simulink model "EV_basic_8_1"  (R2018b)
settings: Solver=VariableStepAuto  StartTime=0.0  StopTime=950  MaxStep=1e-2  MinStep=1e-4  RelTol=1e-2
values from neighbouring files (symbols this model uses):
  Av = 2.75    [InitiateModel.m]    (also in InitiateModel_layouts.m; nurburg_lap.mat)
  batt_max_v = cell_series*cell_max_v    [InitiateModel.m]    (also in nurburg_lap.mat = 613.2)
  Capacity = batt_cap*1e3*3600    (= 252000000)    [InitiateModel.m]    (also in InitiateModel_layouts.m = 252000; nurburg_lap.mat = 180000000)
  Cd = 0.26    [InitiateModel.m]    (also in InitiateModel_layouts.m; nurburg_lap.mat)
  Cr = 0.01    [InitiateModel.m]    (also in InitiateModel_layouts.m; nurburg_lap.mat)
  eta_DC = .985    (= 0.985)    [InitiateModel.m]    (also in InitiateModel_layouts.m; nurburg_lap.mat)
  eta_inv = .965    (= 0.965)    [InitiateModel.m]    (also in InitiateModel_layouts.m; nurburg_lap.mat)
  front_motor = 2    [InitiateModel.m]    (also in nurburg_lap.mat = 0)
  Fv_max = 2*Fv_max_electric    (= 22377.6223776)    [InitiateModel.m]    (also in InitiateModel_layouts.m = 16783.2167832; nurburg_lap.mat)
  Fz_tire = (Mv * weight_dist * 0.5)*9.81    [InitiateModel.m]    (also in nurburg_lap.mat = 5290.7414625)
  gratio = 7    [InitiateModel.m]    (also in InitiateModel_layouts.m = 5.3; nurburg_lap.mat = 5.5)
  grav = 9.81    [InitiateModel.m]    (also in InitiateModel_layouts.m; nurburg_lap.mat)
  inv_eff = 0.98    [InitiateModel.m]    (also in nurburg_lap.mat)
  Ke = 0.607    [InitiateModel.m]    (also in InitiateModel_layouts.m; nurburg_lap.mat)
  max_curr = cell_max_curr*cells_parallel    [InitiateModel.m]    (also in InitiateModel_layouts.m = 270; nurburg_lap.mat = 400)
  motoreff_T = linspace(0,300,101)    [InitiateModel.m]    (also in motoreff_w.mat = [0 4 8 12 16 20 24 28 32 36 40 44 ... (101 elements, 1x101)]; nurburg_lap.mat = [0 3 6 9 12 15 18 21 24 27 30 33 ... (101 elements, 1x101)])
  motoreff_w = [0 18 36 54 72 90 108 126 144 162 180 198 ... (101 elements, 1x101)]    [motoreff_w.mat]    (also in nurburg_lap.mat = [0 12 24 36 48 60 72 84 96 108 120 132 ... (101 elements, 1x)
  Mv = 1420    [InitiateModel.m]    (also in InitiateModel_layouts.m; nurburg_lap.mat)
  opt_slip = 0.18    [InitiateModel.m]    (also in nurburg_lap.mat)
  Pe_max = 160e3    (= 160000)    [InitiateModel.m]    (also in InitiateModel_layouts.m = 120000; nurburg_lap.mat)
  rear_motor = 2    [InitiateModel.m]    (also in nurburg_lap.mat)
  regen_eff = 0.8    [InitiateModel.m]    (also in nurburg_lap.mat)
  rho_air = 1.204    [InitiateModel.m]    (also in InitiateModel_layouts.m; nurburg_lap.mat)
  rw = 0.668/2    (= 0.334)    [InitiateModel.m]    (also in InitiateModel_layouts.m; nurburg_lap.mat)
  s_time = 0.01    [InitiateModel.m]    (also in InitiateModel_layouts.m; nurburg_lap.mat)
  SOC_0 = 80    [InitiateModel.m]    (also in InitiateModel_layouts.m; nurburg_lap.mat)
  Te_max = 2*Te_max_electric    (= 2442.52479547)    [InitiateModel.m]    (also in InitiateModel_layouts.m = 1831.8935966; nurburg_lap.mat)
  tstep = .01    (= 0.01)    [InitiateModel.m]    (also in InitiateModel_layouts.m; nurburg_lap.mat)
  Vbase = 14.30    (= 14.3)    [InitiateModel.m]    (also in InitiateModel_layouts.m; nurburg_lap.mat)
  Vbus_ref = 600    [InitiateModel.m]    (also in InitiateModel_layouts.m = 530; nurburg_lap.mat)
  W_d = 0.5    [InitiateModel.m]    (also in InitiateModel_layouts.m; nurburg_lap.mat)
undefined symbols (not defined in the file or in its folder): MException, throw
libraries: simulink x6, autolibshared x3, peGeneralControl x1, autolibdcdc x1
(part 1 of 4)
settings Model: PacingRate=112  Creator=ignaciovicente  LastModifiedBy=htpc
settings SolverCC: ZeroCrossAlgorithm=Adaptive
settings OptimizationCC: EfficientMapNaN2IntZero=off
settings DebuggingCC: MaskedZcDiagnostic=none  IgnoredZcDiagnostic=none  LibraryContextMissingDiagnostic=none
settings HardwareCC: ProdBitPerLong=64  ProdHWDeviceType=Intel->x86-64 (Mac OS X)  TargetBitPerPointer=64  TargetBitPerSizeT=64  TargetBitPerPtrDiffT=64  TargetLongLongMode=on  TargetIntDivRoundTo=Zero  TargetEndianess=LittleEndian  TargetWordSize=64  TargetHWDeviceType=MATLAB Host  ProdEqTarget=off
settings SFSimCC: SimUseLocalCustomCode=off
settings CodeAppCC: MaxIdLength=128
settings GRTTargetCC: TargetLangStandard=C89/C90 (ANSI)  CombineOutputUpdateFcns=off  GRTInterface=on

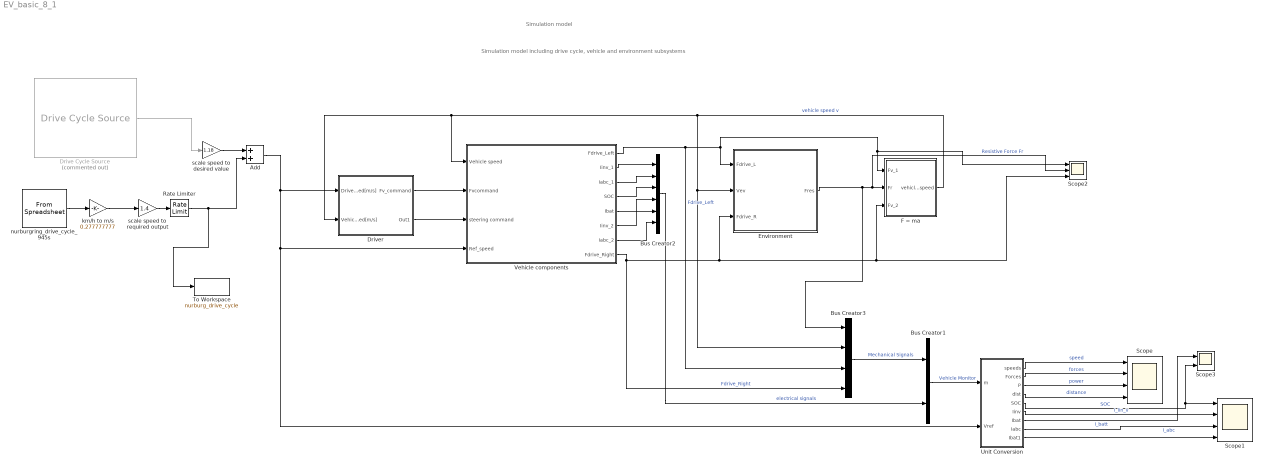
== system EV_basic_8_1 ==
  note: Simulation model including drive cycle, vehicle and environment subsystems
  note: Simulation model
  Add : Sum
  Bus Creator1 : BusCreator  Inputs=2
  Bus Creator2 : BusCreator  Inputs=6
  Bus Creator3 : BusCreator  Inputs=4
  Drive Cycle Source : autolibshared/Drive Cycle Source  Commented=on  cycleVar=FTP75  wsVar=nurburg_time  fileVar=cycleFTP75.mat  tfinal="2474  seconds"  cycleRepeat=off  outAccPort=off  outGearPort=off  gearList=No gear data  t_wot1=5  xdot_woto=0  xdot_wot1=30  t_wot2=30  xdot_wot2=0  t_wotend=40  srcUnit=m/s  outUnit=m/s  srcAccUnit=m/s/s  outAccUnit=m/s^2  dt=0  aMode=1
      settings: SourceProductName=Powertrain Blockset  SourceProductBaseCode=PW
  Driver : Subsystem  AncestorBlock=Driver_Glider_Library/Driver
      mask Display: image('car_driver.jpg');
  "Environment " : Subsystem
      mask Display: image(imread('carretera.jpg'))
  F = ma : Subsystem
  Rate Limiter : RateLimiter  RisingSlewLimit=2  FallingSlewLimit=-2  SampleTimeMode=inherited
  Scope : Scope  NumInputPorts=4
  Scope1 : Scope  NumInputPorts=4
  Scope2 : Scope  NumInputPorts=3
  Scope3 : Scope  NumInputPorts=2
  To Workspace : ToWorkspace  VariableName=nurburg_drive_cycle  SaveFormat=Structure With Time  SampleTime=-1
      settings: Decimation=2
  Unit Conversion : Subsystem
  Vehicle components : Subsystem
      mask Display: image(imread('car_slide.jpg'))
  km/h to m/s : Gain  Gain=0.277777777
  nurburgring_drive_cycle_945s : FromSpreadsheet  FileName=nurburg_data.xlsx  Range=d11:e844  OutDataTypeStr=uint32  SampleTime=s_time
      mask Display: image('/home/ignacio/Dropbox/Q2_2018_19_drop/TFG/models/simulink_modified_Model/images/Circuit_Nurburgring.svg');
  scale speed to desired value : Gain  Gain=1.18
  scale speed to required output : Gain  Gain=1.4
  wires:
  Unit Conversion/1(speeds) -> Scope/1  "speed"
  Bus Creator2/1 -> Bus Creator1/2  "electrical signals"
  Unit Conversion/2(Forces) -> Scope/2  "forces"
  Unit Conversion/5(SOC) -> Scope3/2, Scope1/1  "SOC"
  Unit Conversion/4(dist) -> Scope/4  "distance"
  Vehicle components/5(Ibat) -> Bus Creator2/4
  Bus Creator3/1 -> Bus Creator1/1  "Mechanical Signals"
  Vehicle components/3(Iabc_1) -> Bus Creator2/2
  "Environment "/1(Fres) -> Scope2/2, F = ma/2(Fr), Bus Creator3/1  "Resistive Force Fr"
  Vehicle components/6(Iinv_2) -> Bus Creator2/5
  Vehicle components/4(SOC) -> Bus Creator2/3
  Unit Conversion/8(Iabc) -> Scope1/3  "I_abc"
  Vehicle components/2(Iinv_1) -> Bus Creator2/1
  Vehicle components/1("Fdrive_Left ") -> Bus Creator3/3, Scope2/1, F = ma/1(Fv_1), "Environment "/1(Fdrive_L)  "Fdrive_Left"
  Unit Conversion/3(P) -> Scope/3  "power"
  F = ma/1(vehicle_speed) -> Driver/2(VehicleSpeed[m/s]), Vehicle components/1(Vehicle speed), Bus Creator3/2, "Environment "/2(Vev)  "vehicle speed v"
  Vehicle components/8("Fdrive_Right ") -> Bus Creator3/4, "Environment "/3(Fdrive_R), Scope2/3, F = ma/3(Fv_2)  "Fdrive_Right"
  Vehicle components/7(Iabc_2) -> Bus Creator2/6
  Add/1 -> Unit Conversion/2(Vref), Vehicle components/4(Ref_speed), Driver/1(DriveCycleSpeed[m/s])
  Bus Creator1/1 -> Unit Conversion/1(m)  "Vehicle Monitor"
  Driver/1(Fv_command) -> Vehicle components/2(Fvcommand)
  Driver/2(Out1) -> Vehicle components/3(steering command)
  nurburgring_drive_cycle_945s/1 -> km/h to m/s/1
  Drive Cycle Source/1 -> scale speed to desired value/1
  km/h to m/s/1 -> scale speed to required output/1
  Unit Conversion/9(Ibat1) -> Scope1/4
  Unit Conversion/6(Iinv) -> Scope1/2  "I_lin_v"
  Unit Conversion/7(Ibat) -> Scope3/1  "I_batt"
  scale speed to required output/1 -> Rate Limiter/1
  Rate Limiter/1 -> To Workspace/1, Add/2
  scale speed to desired value/1 -> Add/1

== system EV_basic_8_1/Driver ==
  note: Driver Model
  note: Driver is given PI dynamics to control vehicle speed to a given reference.
      | Output control value is drvier's input to vehicle via gas pedal
  DriveCycleSpeed[m/s] : Inport
  VehicleSpeed[m/s] : Inport  Port=2
  Control error : Scope  NumInputPorts=3
  Max Force Command limiter : Saturate  UpperLimit=Fv_max*12  LowerLimit=-Fv_max*2
  PID Controller : simulink/Continuous/PID Controller  Controller=PID  Form=Parallel  TimeDomain=Continuous-time  SampleTime=-1  IntegratorMethod=Forward Euler  FilterMethod=Forward Euler  ControllerParametersSource=internal  P=1800  I=20  D=0  UseFilter=on  N=0  TunerSelectOption=Transfer Function Based (PID Tuner App)  InitialConditionSource=internal  InitialConditionForIntegrator=0  InitialConditionForFilter=0  DifferentiatorICPrevScaledInput=0  ExternalReset=none  TrackingMode=off  Kt=1  LimitOutput=on  UpperSaturationLimit=Fv_max  LowerSaturationLimit=-Fv_max  LinearizeAsGain=on  AntiWindupMode=none  Kb=1  POutMin=[]  POutMax=[]  IOutMin=[]  IOutMax=[]  DOutMin=[]  DOutMax=[]  NOutMin=[]  NOutMax=[]  SumOutMin=[]  SumOutMax=[]  SaturationOutMin=[]  SaturationOutMax=[]  PParamMin=[]  PParamMax=[]  IParamMin=[]  IParamMax=[]  DParamMin=[]  DParamMax=[]  NParamMin=[]  NParamMax=[]  KbParamMin=[]  KbParamMax=[]  KtParamMin=[]  KtParamMax=[]  KbOutMin=[]  KbOutMax=[]  KtOutMin=[]  KtOutMax=[]  IntegratorOutMin=[]  IntegratorOutMax=[]  FilterOutMin=[]  FilterOutMax=[]  SumI1OutMin=[]  SumI1OutMax=[]  SumI2OutMin=[]  SumI2OutMax=[]  SumI3OutMin=[]  SumI3OutMax=[]  SumI4OutMin=[]  SumI4OutMax=[]  SumDOutMin=[]  SumDOutMax=[]  DifferentiatorOutMin=[]  DifferentiatorOutMax=[]  FilterDiffOutCoefMin=[]  FilterDiffOutCoefMax=[]  ReciprocalOutMin=[]  ReciprocalOutMax=[]  SumDenOutMin=[]  SumDenOutMax=[]  SumNumOutMin=[]  SumNumOutMax=[]  DivideOutMin=[]  DivideOutMax=[]  IntegratorContinuousStateAttributes=''  IntegratorStateMustResolveToSignalObject=off  IntegratorRTWStateStorageClass=Auto  FilterContinuousStateAttributes=''  FilterStateMustResolveToSignalObject=off  FilterRTWStateStorageClass=Auto  ParallelPVariant=InternalParameters  IdealPVariant=Disabled  IVariant=InternalParameters  DVariant=InternalParameters  IntegratorVariant=Continuous  SatVariant=Enabled  AWVariant=Passthrough  PCopyVariant=Disabled  TRVariant=Disabled  FdbkBlocksVariant=Forward  IdealPFdbkVariant=Disabled  SatFdbkVariant=Disabled  DerivativeFilterVariant=ContFilter  NVariant=InternalParameters  NCopyVariant=Disabled  FilterICVariant=InternalICsFilter  IntegratorICVariant=InternalICs  ExternalResetVariant=Disabled  TRSumVariant=Passthrough  SumFdbkVariant=Disabled  SumVariant=Sum_PID
  Sum : Sum  Inputs=+-
  Uniform Random Number : UniformRandomNumber  Minimum=-90  Maximum=90  SampleTime=1
  Fv_command : Outport
  Out1 : Outport  Port=2
  wires:
  Sum/1 -> Control error/1, PID Controller/1  "Error[m/s]"
  VehicleSpeed[m/s]/1 -> Control error/3, Sum/2
  DriveCycleSpeed[m/s]/1 -> Control error/2, Sum/1
  PID Controller/1 -> Max Force Command limiter/1  "DriverCommand"
  Max Force Command limiter/1 -> Fv_command/1
  Uniform Random Number/1 -> Out1/1

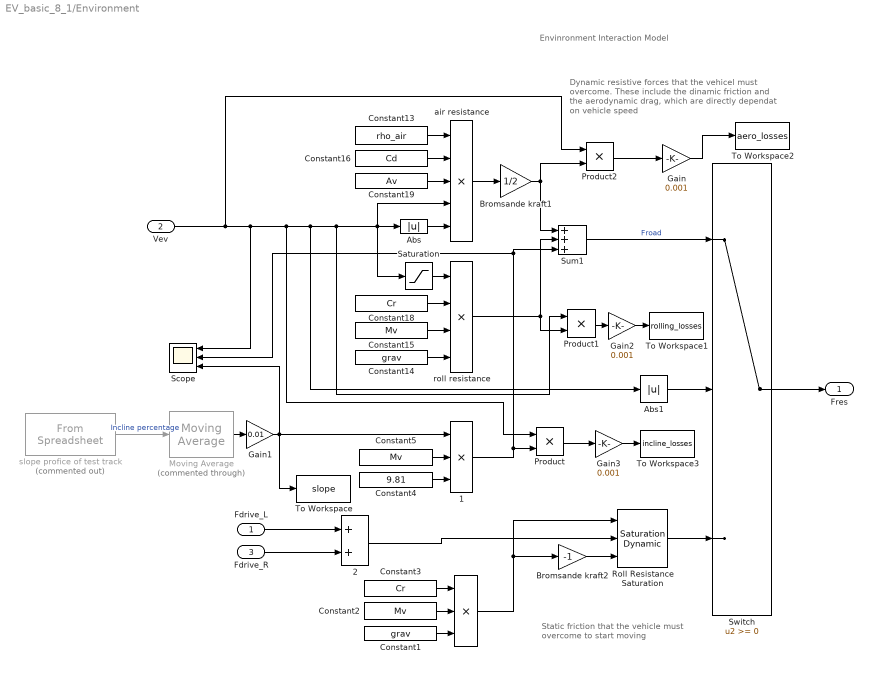
== system EV_basic_8_1/Environment  ==
  note: Static friction that the vehicle must overcome to start moving
  note: Dynamic resistive forces that the vehicel must overcome. These include the dinamic friction and the aerodynamic drag, which are directly dependat on vehicle speed
  note: Envinronment Interaction Model
  Fdrive_L : Inport
  Vev : Inport  Port=2
  Fdrive_R : Inport  Port=3
  "   " : Product  Inputs=3  SaturateOnIntegerOverflow=on  InputSameDT=on  OutDataTypeStr=Inherit: Same as first input
  "   1" : Product  Inputs=3  SaturateOnIntegerOverflow=on  InputSameDT=on  OutDataTypeStr=Inherit: Same as first input
  "   2" : Sum
  Abs : Abs  SaturateOnIntegerOverflow=on
  Abs1 : Abs
  Bromsande kraft1 : Gain  Gain=1/2  SaturateOnIntegerOverflow=on  OutDataTypeStr=Inherit: Same as input  ParamDataTypeStr=Inherit: Same as input
  Bromsande kraft2 : Gain  Gain=-1  SaturateOnIntegerOverflow=on  OutDataTypeStr=Inherit: Same as input  ParamDataTypeStr=Inherit: Same as input
  Constant1 : Constant  Value=grav
  Constant13 : Constant  Value=rho_air
  Constant14 : Constant  Value=grav
  Constant15 : Constant  Value=Mv
  Constant16 : Constant  Value=Cd
  Constant18 : Constant  Value=Cr
  Constant19 : Constant  Value=Av
  Constant2 : Constant  Value=Mv
  Constant3 : Constant  Value=Cr
  Constant4 : Constant  Value=9.81
  Constant5 : Constant  Value=Mv
  Gain : Gain  Gain=0.001
  Gain1 : Gain  Gain=0.01
  Gain2 : Gain  Gain=0.001
  Gain3 : Gain  Gain=0.001
  Moving Average : peGeneralControl/Moving Average  Commented=through  VariantControl=Variant1  LabelModeActiveChoice=Discrete  f=20  x0=0  Ts=-1
  Product : Product
  Product1 : Product
  Product2 : Product
  Roll Resistance Saturation : simulink/Discontinuities/Saturation Dynamic  OutMin=[]  OutMax=[]  OutDataTypeStr=Inherit: Same as second input  OutDataType=fixdt(1, 16)  OutScaling=2^-10  DoSatur=off
  Saturation : Saturate  UpperLimit=1  LowerLimit=-1
  Scope : Scope  NumInputPorts=3
  Sum1 : Sum  Inputs=+++  SaturateOnIntegerOverflow=on  InputSameDT=on  OutDataTypeStr=Inherit: Same as first input
  Switch : Switch
  To Workspace : ToWorkspace  VariableName=slope  SaveFormat=Structure With Time  SampleTime=s_time
  To Workspace1 : ToWorkspace  VariableName=rolling_losses  SaveFormat=Structure With Time  SampleTime=s_time
  To Workspace2 : ToWorkspace  VariableName=aero_losses  SaveFormat=Structure With Time  SampleTime=s_time
  To Workspace3 : ToWorkspace  VariableName=incline_losses  SaveFormat=Structure With Time  SampleTime=s_time
  air resistance : Product  Inputs=5  SaturateOnIntegerOverflow=on  InputSameDT=on  OutDataTypeStr=Inherit: Same as first input
  roll resistance : Product  Inputs=4  SaturateOnIntegerOverflow=on  InputSameDT=on  OutDataTypeStr=Inherit: Same as first input
  slope profice of test track : FromSpreadsheet  Commented=on  FileName=nurburg_data.xlsx  Range=d11:d844, i11:i844  SampleTime=s_time
  Fres : Outport  InitialOutput=0
  wires:
  air resistance/1 -> Bromsande kraft1/1
  Bromsande kraft1/1 -> Sum1/1, Product2/2
  Constant13/1 -> air resistance/1
  Constant16/1 -> air resistance/2
  Constant19/1 -> air resistance/3
  Constant18/1 -> roll resistance/2
  Constant15/1 -> roll resistance/3
  Constant14/1 -> roll resistance/4
  Abs/1 -> air resistance/5
  Saturation/1 -> roll resistance/1
  Sum1/1 -> Switch/1  "Froad"
  Vev/1 -> Product2/1, Product/1, Abs1/1, Product1/1, air resistance/4, Saturation/1, Abs/1, Scope/1
  roll resistance/1 -> Product1/2, Sum1/2
  Roll Resistance Saturation/1 -> Switch/3
  Abs1/1 -> Switch/2
  Constant3/1 -> "   "/1
  Constant2/1 -> "   "/2
  Constant1/1 -> "   "/3
  "   "/1 -> Roll Resistance Saturation/1, Bromsande kraft2/1
  Bromsande kraft2/1 -> Roll Resistance Saturation/3
  Constant5/1 -> "   1"/2
  Constant4/1 -> "   1"/3
  "   1"/1 -> Product/2, Scope/2, Sum1/3
  slope profice of test track/1 -> Moving Average/1  "Incline percentage"
  Gain1/1 -> To Workspace/1, Scope/3, "   1"/1
  Fdrive_L/1 -> "   2"/1
  Fdrive_R/1 -> "   2"/2
  "   2"/1 -> Roll Resistance Saturation/2
  Switch/1 -> Fres/1
  Gain/1 -> To Workspace2/1
  Gain3/1 -> To Workspace3/1
  Gain2/1 -> To Workspace1/1
  Product1/1 -> Gain2/1
  Product2/1 -> Gain/1
  Product/1 -> Gain3/1
  Moving Average/1 -> Gain1/1

== system EV_basic_8_1/F = ma ==
  note: Application of Newton's law to calculate vehicle slip from the acting vehicle forces
  note: Newton's law
  Fv_1 : Inport
  Fr : Inport  Port=2
  Fv_2 : Inport  Port=3
  "   " : Sum  Inputs=++-
  Acceleration [m/s^2] to speed [m/s] : Integrator
  Force [N] to acceleration [m/s^2] : Gain  Gain=1/Mv
  vehicle_speed : Outport
  wires:
  "   "/1 -> Force [N] to acceleration [m/s^2]/1  "Net Force"
  Force [N] to acceleration [m/s^2]/1 -> Acceleration [m/s^2] to speed [m/s]/1  "Vehicle Acceleration"
  Fv_1/1 -> "   "/1
  Acceleration [m/s^2] to speed [m/s]/1 -> vehicle_speed/1  "Vehicle Speed"
  Fr/1 -> "   "/3
  Fv_2/1 -> "   "/2

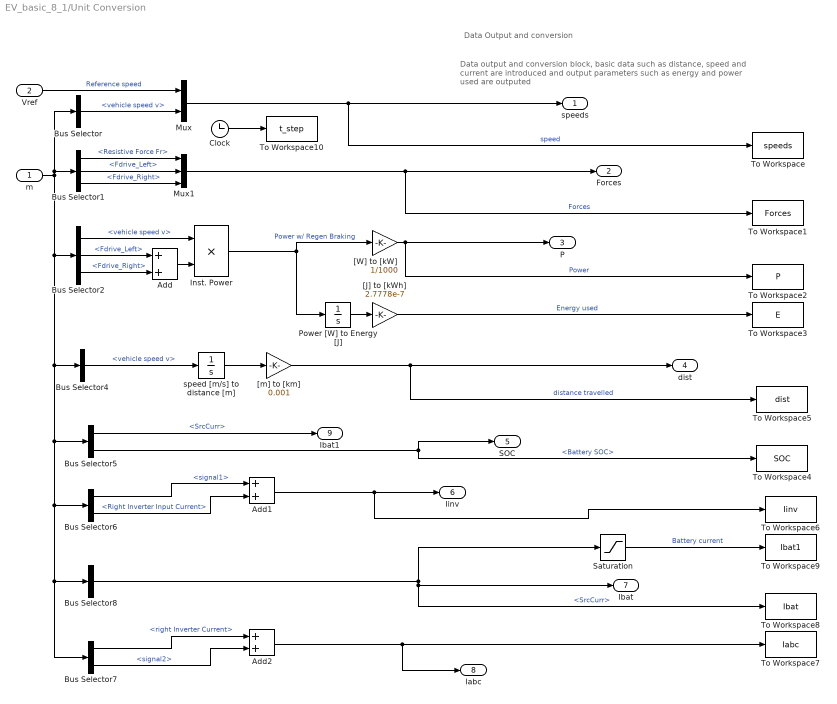
== system EV_basic_8_1/Unit Conversion ==
  note: Data output and conversion block, basic data such as distance, speed
      |  and current are introduced and output parameters such as energy
      | and power used are outputed
  note: Data Output and conversion
  m : Inport
  Vref : Inport  Port=2
  Add : Sum
  Add1 : Sum
  Add2 : Sum
  Bus Selector : BusSelector  OutputSignals=Mechanical Signals.vehicle speed v
  Bus Selector1 : BusSelector  OutputSignals=Mechanical Signals.Resistive Force Fr,Mechanical Signals.Fdrive_Left,Mechanical Signals.Fdrive_Right
  Bus Selector2 : BusSelector  OutputSignals=Mechanical Signals.vehicle speed v,Mechanical Signals.Fdrive_Left,Mechanical Signals.Fdrive_Right
  Bus Selector4 : BusSelector  OutputSignals=Mechanical Signals.vehicle speed v
  Bus Selector5 : BusSelector  OutputSignals=electrical signals.SrcCurr,electrical signals.Battery SOC
  Bus Selector6 : BusSelector  OutputSignals=electrical signals.signal1,electrical signals.Right Inverter Input Current
  Bus Selector7 : BusSelector  OutputSignals=electrical signals.right Inverter Current,electrical signals.signal2
  Bus Selector8 : BusSelector  OutputSignals=electrical signals.SrcCurr
  Clock : Clock
  Inst. Power : Product  RndMeth=Zero
  Mux : Mux  Inputs=2
  Mux1 : Mux  Inputs=3
  Power [W] to Energy [J] : Integrator
  Saturation : Saturate  UpperLimit=1000  LowerLimit=0
  To Workspace : ToWorkspace  VariableName=speeds  SaveFormat=Structure With Time  SampleTime=s_time
  To Workspace1 : ToWorkspace  VariableName=Forces  SaveFormat=Structure With Time  SampleTime=s_time
  To Workspace10 : ToWorkspace  VariableName=t_step  SampleTime=tstep
      settings: Decimation=3  Save2DSignal=2-D array (concatenate along first dimension)
  To Workspace2 : ToWorkspace  VariableName=P  SaveFormat=Structure With Time  SampleTime=s_time
  To Workspace3 : ToWorkspace  VariableName=E  SaveFormat=Structure With Time  SampleTime=s_time
  To Workspace4 : ToWorkspace  VariableName=SOC  SaveFormat=Structure With Time  SampleTime=s_time
      settings: Save2DSignal=2-D array (concatenate along first dimension)
  To Workspace5 : ToWorkspace  VariableName=dist  SaveFormat=Structure With Time  SampleTime=tstep
      settings: Save2DSignal=2-D array (concatenate along first dimension)
  To Workspace6 : ToWorkspace  VariableName=Iinv  SaveFormat=Structure With Time  SampleTime=s_time
  To Workspace7 : ToWorkspace  VariableName=Iabc  SaveFormat=Structure With Time  SampleTime=s_time
  To Workspace8 : ToWorkspace  VariableName=Ibat  SaveFormat=Structure With Time  SampleTime=s_time
  To Workspace9 : ToWorkspace  VariableName=Ibat1  SaveFormat=Structure With Time  SampleTime=s_time
  "[J] to [kWh]" : Gain  Gain=2.7778e-7
  "[W] to [kW]" : Gain  Gain=1/1000
  "[m] to [km]" : Gain  Gain=0.001
  speed [m/s] to distance [m] : Integrator
  speeds : Outport
  Forces : Outport  Port=2
  P : Outport  Port=3
  dist : Outport  Port=4
  SOC : Outport  Port=5
  Iinv : Outport  Port=6
  Ibat : Outport  Port=7
  Iabc : Outport  Port=8
  Ibat1 : Outport  Port=9
  wires:
  m/1 -> Bus Selector/1, Bus Selector1/1, Bus Selector2/1, Bus Selector5/1, Bus Selector6/1, Bus Selector8/1, Bus Selector7/1, Bus Selector4/1
  Mux1/1 -> To Workspace1/1, Forces/1  "Forces"
  Bus Selector2/1 -> Inst. Power/1  "<vehicle speed v>"
  Bus Selector4/1 -> speed [m/s] to distance [m]/1  "<vehicle speed v>"
  speed [m/s] to distance [m]/1 -> "[m] to [km]"/1
  "[m] to [km]"/1 -> dist/1, To Workspace5/1  "distance travelled"
  Bus Selector/1 -> Mux/2  "<vehicle speed v>"
  Vref/1 -> Mux/1  "Reference speed"
  "[W] to [kW]"/1 -> P/1, To Workspace2/1  "Power"
  Power [W] to Energy [J]/1 -> "[J] to [kWh]"/1
  "[J] to [kWh]"/1 -> To Workspace3/1  "Energy used"
  Inst. Power/1 -> "[W] to [kW]"/1, Power [W] to Energy [J]/1  "Power w/ Regen Braking"
  Bus Selector5/2 -> SOC/1, To Workspace4/1  "<Battery SOC>"
  Bus Selector8/1 -> Saturation/1, Ibat/1, To Workspace8/1  "<SrcCurr>"
  Saturation/1 -> To Workspace9/1  "Battery current"
  Mux/1 -> To Workspace/1, speeds/1  "speed"
  Bus Selector2/2 -> Add/1  "<Fdrive_Left>"
  Bus Selector2/3 -> Add/2  "<Fdrive_Right>"
  Add/1 -> Inst. Power/2
  Bus Selector1/2 -> Mux1/2  "<Fdrive_Left>"
  Bus Selector1/3 -> Mux1/3  "<Fdrive_Right>"
  Bus Selector1/1 -> Mux1/1  "<Resistive Force Fr>"
  Bus Selector6/2 -> Add1/2  "<Right Inverter Input Current>"
  Bus Selector6/1 -> Add1/1  "<signal1>"
  Add1/1 -> To Workspace6/1, Iinv/1
  Bus Selector7/1 -> Add2/1  "<right Inverter Current>"
  Bus Selector7/2 -> Add2/2  "<signal2>"
  Add2/1 -> Iabc/1, To Workspace7/1
  Bus Selector5/1 -> Ibat1/1  "<SrcCurr>"
  Clock/1 -> To Workspace10/1

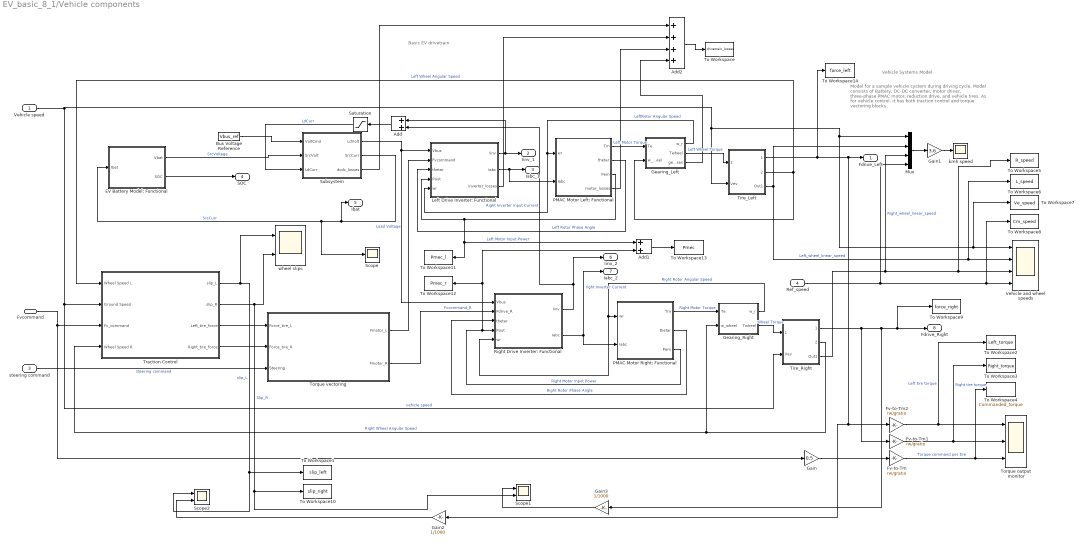
== system EV_basic_8_1/Vehicle components ==
  note: Basic EV drivetrain
  note: Vehicle Systems Model
  note: Model for a sample vehicle system during driving cycle. Model consists
      | of Battery, DC-DC converter, motor driver, three-phase PMAC motor, reduction drive, and vehicle tires.
      | As for vehicle control, it has both traction control and torque vectoring blocks
  Vehicle speed : Inport
  Fvcommand : Inport  Port=2
  steering command : Inport  Port=3
  Ref_speed : Inport  Port=4
  Add : Sum
  Add1 : Sum
  Add2 : Sum  Inputs=++++
  Bus Voltage Reference : Constant  Value=Vbus_ref
  EV Battery Model: Functional : Subsystem
      mask Display: image(imread('batt_pack.jpg'))
  Fv-to-Tm : Gain  Gain=rw/gratio
  Fv-to-Tm1 : Gain  Gain=rw/gratio
  Fv-to-Tm2 : Gain  Gain=rw/gratio
  Gain : Gain  Gain=0.5
  Gain1 : Gain  Gain=3.6
  Gain2 : Gain  Gain=1/1000
  Gain3 : Gain  Gain=1/1000
  Gearing_Left : Subsystem
      mask Display: image(imread('gearbox.jpg'))
  Gearing_Right : Subsystem
      mask Display: image(imread('gearbox.jpg'))
  Left Drive Inverter: Functional : Subsystem
      mask Display: image(imread('inverter.jpg'))
  Mux : Mux
  PMAC Motor Left: Functional : Subsystem
      mask Display: image(imread('electric_motor.jpg'))
  PMAC Motor Right: Functional : Subsystem
      mask Display: image(imread('electric_motor.jpg'))
  Right Drive Inverter: Functional : Subsystem
      mask Display: image(imread('inverter.jpg'))
  Saturation : Saturate  UpperLimit=333  LowerLimit=-333
  Scope : Scope
  Scope1 : Scope  NumInputPorts=2
  Scope2 : Scope  NumInputPorts=2
  Subsystem : Subsystem
      mask Display: image('/home/ignacio/Pictures/Screenshot from 2019-05-29 11-25-46.png');
  Tire_Left : Subsystem
      mask Display: image(imread('car_wheel.png'))
  Tire_Right : Subsystem
      mask Display: image(imread('car_wheel.png'))
  To Workspace : ToWorkspace  VariableName=drivetrain_losses  SaveFormat=Structure With Time  SampleTime=s_time
  To Workspace1 : ToWorkspace  VariableName=slip_left  SaveFormat=Structure With Time  SampleTime=s_time
  To Workspace10 : ToWorkspace  VariableName=slip_right  SaveFormat=Structure With Time  SampleTime=s_time
  To Workspace11 : ToWorkspace  VariableName=Pmec_l  SaveFormat=Structure With Time  SampleTime=s_time
  To Workspace12 : ToWorkspace  VariableName=Pmec_r  SaveFormat=Timeseries  SampleTime=s_time
  To Workspace13 : ToWorkspace  VariableName=Pmec  SaveFormat=Structure With Time  SampleTime=s_time
  To Workspace14 : ToWorkspace  VariableName=force_left  SaveFormat=Structure With Time  SampleTime=s_time
  To Workspace2 : ToWorkspace  VariableName=Left_torque  SaveFormat=Structure With Time  SampleTime=tstep
  To Workspace3 : ToWorkspace  VariableName=Right_torque  SaveFormat=Structure With Time  SampleTime=tstep
  To Workspace4 : ToWorkspace  VariableName=Commanded_torque  SaveFormat=Structure With Time  SampleTime=tstep
  To Workspace5 : ToWorkspace  VariableName=R_speed  SaveFormat=Structure With Time  SampleTime=tstep
  To Workspace6 : ToWorkspace  VariableName=L_speed  SaveFormat=Structure With Time  SampleTime=tstep
  To Workspace7 : ToWorkspace  VariableName=Ve_speed  SaveFormat=Structure With Time  SampleTime=tstep
  To Workspace8 : ToWorkspace  VariableName=Cm_speed  SaveFormat=Structure With Time  SampleTime=tstep
  To Workspace9 : ToWorkspace  VariableName=force_right  SaveFormat=Structure With Time  SampleTime=s_time
  Torque output monitor : Scope  NumInputPorts=3
  Torque vectoring : Subsystem
      mask Display: image(imread('torque_vectoring.jpg'))
  Traction Control : Subsystem
      mask Display: image(imread('traction_control.png'))
  Vehicle and wheel speeds : Scope  NumInputPorts=4
  kmh speed : Scope
  wheel slips : Scope  NumInputPorts=2
  "Fdrive_Left " : Outport
  Iinv_1 : Outport  Port=2
  Iabc_1 : Outport  Port=3
  SOC : Outport  Port=4
  Ibat : Outport  Port=5
  Iinv_2 : Outport  Port=6
  Iabc_2 : Outport  Port=7
  "Fdrive_Right " : Outport  Port=8
  wires:
  EV Battery Model: Functional/1(Vbat) -> Subsystem/2(SrcVolt)  "SrcVoltage"
  Subsystem/2(SrcCurr) -> Scope/1, EV Battery Model: Functional/1(Ibat), Ibat/1  "SrcCurr"
  EV Battery Model: Functional/2(SOC) -> SOC/1
  Left Drive Inverter: Functional/2(Iabc) -> PMAC Motor Left: Functional/2(Iabc), Iabc_1/1
  Bus Voltage Reference/1 -> Subsystem/1(VoltCmd)
  PMAC Motor Left: Functional/2(thetar) -> Left Drive Inverter: Functional/3(thetar)  "Left Rotor Phase Angle"
  Left Drive Inverter: Functional/1(Iinv) -> Add/1, Iinv_1/1
  Subsystem/1(LdVolt) -> Right Drive Inverter: Functional/1(Vbus), Left Drive Inverter: Functional/1(Vbus)  "Load Voltage"
  PMAC Motor Left: Functional/3(Pem) -> To Workspace11/1, Add1/1, Left Drive Inverter: Functional/4(Pout)  "Left Motor Input Power"
  Tire_Left/1(Fdrive_L) -> Gain2/1, Fv-to-Tm2/1, "Fdrive_Left "/1, To Workspace14/1
  Gearing_Left/2(Twheel) -> Tire_Left/1(Twheel_L)  "Left Wheel Torque"
  Tire_Left/2(Left_wheel_speed) -> Gearing_Left/2(w_wheel), Traction Control/1(Wheel Speed L)  "Left Wheel Angular Speed"
  Gearing_Left/1(w_r) -> PMAC Motor Left: Functional/1(wr), Left Drive Inverter: Functional/5(wr)  "LeftRotor Angular Speed"
  Torque vectoring/1(Fmotor_L) -> Left Drive Inverter: Functional/2(Fvcommand)
  PMAC Motor Left: Functional/1(Tm) -> Gearing_Left/1(Te)  "Left Motor Torque"
  Gearing_Right/2(Twheel) -> Tire_Right/1(Twheel_R)  "Wheel Torque"
  Tire_Right/2(Right_wheel_speed) -> Traction Control/4(Wheel Speed R), Gearing_Right/2(w_wheel)  "Right Wheel Angular Speed"
  PMAC Motor Right: Functional/1(Tm) -> Gearing_Right/1(Te)  "Right Motor Torque"
  PMAC Motor Right: Functional/2(thetar) -> Right Drive Inverter: Functional/3(thetar)  "Right Rotor Phase Angle"
  Right Drive Inverter: Functional/2(Iabc) -> PMAC Motor Right: Functional/2(Iabc), Iabc_2/1  "right Inverter Current"
  Gearing_Right/1(w_r) -> PMAC Motor Right: Functional/1(wr), Right Drive Inverter: Functional/5(wr)  "Right Rotor Angular Speed"
  PMAC Motor Right: Functional/3(Pem) -> Add1/2, To Workspace12/1, Right Drive Inverter: Functional/4(Pout)  "Right Motor Input Power"
  Right Drive Inverter: Functional/1(Iinv) -> Add/2, Iinv_2/1  "Right Inverter Input Current"
  Torque vectoring/2(Fmotor_R) -> Right Drive Inverter: Functional/2(Fdrive_R)  "Fvcommand_R"
  Fvcommand/1 -> Gain/1, Traction Control/3(Fv_command)
  Traction Control/3(Left_tire_force) -> Torque vectoring/1(Force_tire_L)
  Vehicle speed/1 -> Tire_Left/2(Vev), Mux/1, To Workspace7/1, Vehicle and wheel speeds/1, Tire_Right/2(Vev), Traction Control/2(Ground Speed)  "vehicle speed"
  steering command/1 -> Torque vectoring/3(Steering)  "steering command"
  Traction Control/1(slip_L) -> Scope2/1, To Workspace1/1, wheel slips/1  "slip_L"
  Traction Control/2(slip_R) -> Scope1/2, To Workspace10/1, wheel slips/2  "Slip_R"
  Traction Control/4(Right_tire_force) -> Torque vectoring/2(Force_tire_R)
  Tire_Right/1(Fdrive_R) -> Fv-to-Tm1/1, Gain3/1, To Workspace9/1, "Fdrive_Right "/1
  Tire_Right/3(Out1) -> Mux/3, To Workspace5/1, Vehicle and wheel speeds/3  "Right_wheel_linear_speed"
  Tire_Left/3(Out1) -> To Workspace6/1, Vehicle and wheel speeds/2, Mux/2  "Left_wheel_linear_speed"
  Ref_speed/1 -> Mux/4, To Workspace8/1, Vehicle and wheel speeds/4
  Fv-to-Tm/1 -> To Workspace4/1, Torque output monitor/3  "Torque command per tire"
  Fv-to-Tm1/1 -> Torque output monitor/2, To Workspace3/1  "Right tire torque"
  Fv-to-Tm2/1 -> To Workspace2/1, Torque output monitor/1  "Left tire torque"
  Gain/1 -> Fv-to-Tm/1
  Mux/1 -> Gain1/1
  Gain1/1 -> kmh speed/1
  Saturation/1 -> Subsystem/3(LdCurr)  "LdCurr"
  Add/1 -> Saturation/1
  Gain2/1 -> Scope2/2
  Gain3/1 -> Scope1/1
  Add1/1 -> To Workspace13/1
  Gearing_Left/3(gearbox_losses) -> Add2/4
  PMAC Motor Left: Functional/4(motor_losses) -> Add2/3
  Left Drive Inverter: Functional/3(inverter_losses) -> Add2/2
  Subsystem/3(dcdc_losses) -> Add2/1
  Add2/1 -> To Workspace/1

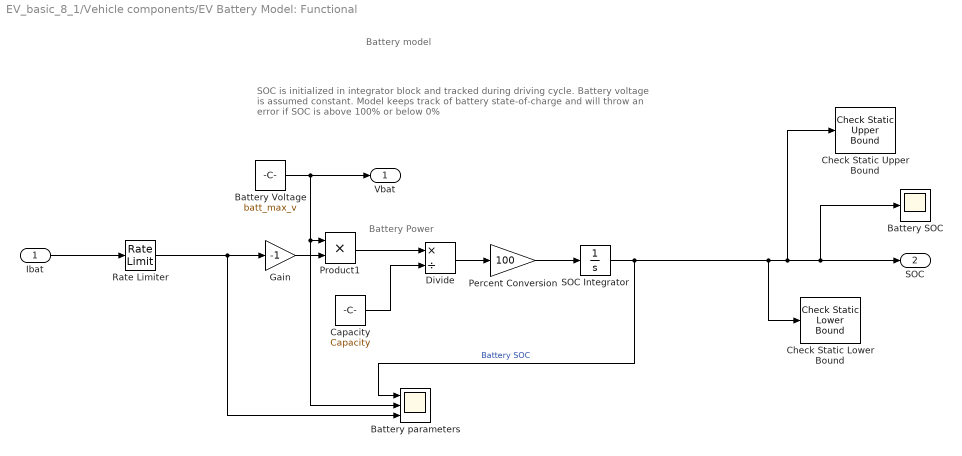
== system EV_basic_8_1/Vehicle components/EV Battery Model: Functional ==
  note: Battery model
  note: Battery
      | Power
  note: SOC is initialized in integrator block and tracked during driving cycle.  Battery
      | voltage is assumed constant.  Model keeps track of battery state-of-charge and
      | will throw an error if SOC is above 100% or below 0%
  Ibat : Inport
  Battery Voltage : Constant  Value=batt_max_v
  "Battery SOC " : Scope
  Battery parameters : Scope  NumInputPorts=3
  Capacity : Constant  Value=Capacity
  Check Static Lower Bound : simulink/Model Verification/Check Static  Lower Bound  Description=0 <= u  min=0  min_included=on  enabled=on  callback=throw(MException('ResultChk:OutOfRange','Battery SOC has fallen below 0'))  stopWhenAssertionFail=on  export=off  icon=graphic
      settings: SourceProductName=Simulink
  Check Static Upper Bound : simulink/Model Verification/Check Static  Upper Bound  Description=u <= 100  max=100  max_included=on  enabled=on  callback=throw(MException('ResultChk:OutOfRange','Battery SOC has exceeded 100'))  stopWhenAssertionFail=on  export=off  icon=graphic
      settings: SourceProductName=Simulink  SourceProductBaseCode=SL
  Divide : Product  Inputs=*/
  Gain : Gain  Gain=-1
  Percent Conversion : Gain  Gain=100
  Product1 : Product  RndMeth=Zero
  Rate Limiter : RateLimiter  RisingSlewLimit=3  FallingSlewLimit=-3  SampleTimeMode=inherited
  SOC Integrator : Integrator  InitialCondition=SOC_0  ZeroCross=off
  Vbat : Outport
  SOC : Outport  Port=2
  wires:
  Ibat/1 -> Rate Limiter/1
  Product1/1 -> Divide/1
  SOC Integrator/1 -> Battery parameters/1, Check Static Upper Bound/1, "Battery SOC "/1, SOC/1, Check Static Lower Bound/1  "Battery SOC"
  Battery Voltage/1 -> Battery parameters/2, Product1/1, Vbat/1
  Gain/1 -> Product1/2
  Capacity/1 -> Divide/2
  Divide/1 -> Percent Conversion/1
  Percent Conversion/1 -> SOC Integrator/1
  Rate Limiter/1 -> Battery parameters/3, Gain/1

== system EV_basic_8_1/Vehicle components/Gearing_Left ==
  note: Model of connection between motor and wheel.  In this
      | example, it is assumed that motor and wheel are directly coupled
      | by an ideal, lossless shaft with no gear reduction.
  note: Vehicle Transmission Model
  Te : Inport
  w_wheel : Inport  Port=2
  Constant : Constant  Value=gratio
  Constant1 : Constant  Value=0.03
  Product : Product  RndMeth=Zero
  Product1 : Product  RndMeth=Zero
  Product2 : Product  Inputs=3
  To Workspace : ToWorkspace  VariableName=gearbox_losses  SaveFormat=Structure With Time  SampleTime=s_time
  geartrain losses : Gain  Gain=0.97
  w_r : Outport
  Twheel : Outport  Port=2
  gearbox_losses : Outport  Port=3
  wires:
  w_wheel/1 -> Product1/2
  Product/1 -> geartrain losses/1
  Constant/1 -> Product/2, Product1/1
  Product2/1 -> gearbox_losses/1, To Workspace/1
  Product1/1 -> Product2/2, w_r/1
  Constant1/1 -> Product2/3
  Te/1 -> Product2/1, Product/1
  geartrain losses/1 -> Twheel/1

== system EV_basic_8_1/Vehicle components/Gearing_Right ==
  note: Model of connection between motor and wheel.  In this
      | example, it is assumed that motor and wheel are directly coupled
      | by an ideal, lossless shaft with no gear reduction.
  note: Vehicle Transmission Model
  Te : Inport
  w_wheel : Inport  Port=2
  Constant : Constant  Value=gratio
  Constant1 : Constant  Value=0.03
  Gain : Gain  Gain=0.97
  Product : Product  RndMeth=Zero
  Product1 : Product  RndMeth=Zero
  Product2 : Product  Inputs=3
  To Workspace : ToWorkspace  VariableName=gearbox_losses_r  SaveFormat=Structure With Time  SampleTime=s_time
  w_r : Outport
  Twheel : Outport  Port=2
  wires:
  Te/1 -> Product2/1, Product/1
  w_wheel/1 -> Product1/2
  Product/1 -> Gain/1
  Product1/1 -> Product2/2, w_r/1
  Constant/1 -> Product/2, Product1/1
  Constant1/1 -> Product2/3
  Gain/1 -> Twheel/1
  Product2/1 -> To Workspace/1

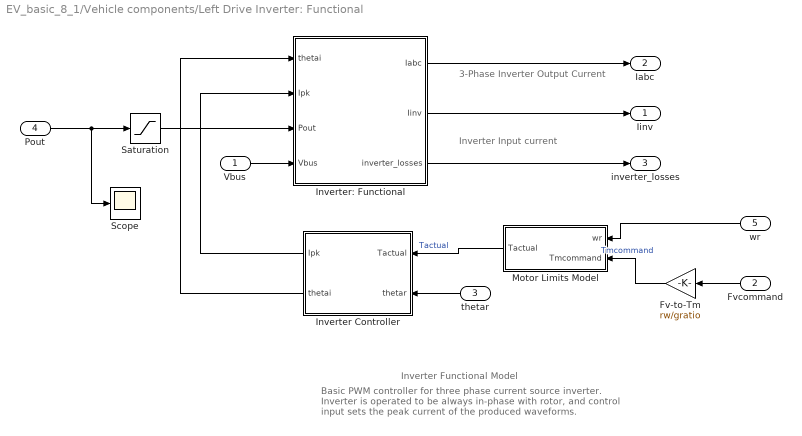
== system EV_basic_8_1/Vehicle components/Left Drive Inverter: Functional ==
  note: 3-Phase Inverter Output Current
  note: Inverter Input current
  note: Basic PWM controller for three phase current source inverter.
      | Inverter is operated to be always in-phase with rotor,
      | and control input sets the peak current of the produced
      | waveforms.
  note: Inverter Functional Model
  Vbus : Inport
  Fvcommand : Inport  Port=2
  thetar : Inport  Port=3
  Pout : Inport  Port=4
  wr : Inport  Port=5
  Fv-to-Tm : Gain  Gain=rw/gratio
  Inverter Controller : Subsystem
  Inverter: Functional : Subsystem
  Motor Limits Model : Subsystem
  Saturation : Saturate  UpperLimit=3e5  LowerLimit=-3e5
  Scope : Scope
  Iinv : Outport
  Iabc : Outport  Port=2
  inverter_losses : Outport  Port=3
  wires:
  Inverter Controller/2(thetai) -> Inverter: Functional/1(thetai)
  Inverter Controller/1(Ipk) -> Inverter: Functional/2(Ipk)
  Inverter: Functional/2(Iinv) -> Iinv/1
  Inverter: Functional/1(Iabc) -> Iabc/1
  thetar/1 -> Inverter Controller/2(thetar)
  Pout/1 -> Scope/1, Saturation/1
  Vbus/1 -> Inverter: Functional/4(Vbus)
  Motor Limits Model/1(Tactual) -> Inverter Controller/1(Tactual)  "Tactual"
  wr/1 -> Motor Limits Model/1(wr)
  Fvcommand/1 -> Fv-to-Tm/1
  Fv-to-Tm/1 -> Motor Limits Model/2(Tmcommand)  "Tmcommand"
  Saturation/1 -> Inverter: Functional/3(Pout)
  Inverter: Functional/3(inverter_losses) -> inverter_losses/1

== system EV_basic_8_1/Vehicle components/PMAC Motor Left: Functional ==
  note: Permanent Magnet AC Motor model is given according to the
      | Torque balance equation, with damping included.  Load torque is supplied
      | externally.  Motor input power is calculated from current speed and torque
      | through efficiency tables provided in the MotorEff.mat file
  note: ECEN 5017 PMAC motor
  note: PMAC Motor Model
  note: Motor model receives three-phase input currents from inverter and
      | rotational speed of rotor from gearing.  Motor outputs torque from ideal
      | motor model and electrical power consumption from motor efficiency model
  wr : Inport
  Iabc : Inport  Port=2
  " " : Constant  Value=2*pi
  Demux : Demux  Outputs=3
  Ideal Motor Model : Subsystem
  Modulus : Math  Operator=mod  SaturateOnIntegerOverflow=on
  Motor Efficiency : Subsystem
  angular speed [rad/s] to angle [rad] : Integrator
  Tm : Outport
  thetar : Outport  Port=2
  Pem : Outport  Port=3
  motor_losses : Outport  Port=4
  wires:
  wr/1 -> Motor Efficiency/1(wr), angular speed [rad/s] to angle [rad]/1  "Rotor Angular speed"
  Iabc/1 -> Demux/1  "3-phase Stator Currents"
  Motor Efficiency/1(Pem) -> Pem/1
  Demux/3 -> Ideal Motor Model/3(Ic)
  Demux/2 -> Ideal Motor Model/2(Ib)
  Demux/1 -> Ideal Motor Model/1(Ia)
  Modulus/1 -> Ideal Motor Model/4(pihr), thetar/1  "Rotor Angle"
  angular speed [rad/s] to angle [rad]/1 -> Modulus/1
  Ideal Motor Model/1(Tm) -> Motor Efficiency/2(Tm), Tm/1  "Motor Torque"
  " "/1 -> Modulus/2
  Motor Efficiency/2(motor_losses) -> motor_losses/1

== system EV_basic_8_1/Vehicle components/PMAC Motor Right: Functional ==
  note: Permanent Magnet AC Motor model is given according to the
      | Torque balance equation, with damping included.  Load torque is supplied
      | externally.  Motor input power is calculated from current speed and torque
      | through efficiency tables provided in the MotorEff.mat file
  note: ECEN 5017 PMAC motor
  note: PMAC Motor Model
  note: Motor model receives three-phase input currents from inverter and
      | rotational speed of rotor from gearing.  Motor outputs torque from ideal
      | motor model and electrical power consumption from motor efficiency model
  wr : Inport
  Iabc : Inport  Port=2
  " " : Constant  Value=2*pi
  Demux : Demux  Outputs=3
  Ideal Motor Model : Subsystem
  Modulus : Math  Operator=mod  SaturateOnIntegerOverflow=on
  Motor Efficiency : Subsystem
  angular speed [rad/s] to angle [rad] : Integrator
  Tm : Outport
  thetar : Outport  Port=2
  Pem : Outport  Port=3
  wires:
  wr/1 -> Motor Efficiency/1(wr), angular speed [rad/s] to angle [rad]/1  "Rotor Angular speed"
  Iabc/1 -> Demux/1  "3-phase Stator Currents"
  Motor Efficiency/1(Pem) -> Pem/1
  Demux/3 -> Ideal Motor Model/3(Ic)
  Demux/2 -> Ideal Motor Model/2(Ib)
  Demux/1 -> Ideal Motor Model/1(Ia)
  Modulus/1 -> Ideal Motor Model/4(pihr), thetar/1  "Rotor Angle"
  angular speed [rad/s] to angle [rad]/1 -> Modulus/1
  Ideal Motor Model/1(Tm) -> Tm/1, Motor Efficiency/2(Tm)  "Motor Torque"
  " "/1 -> Modulus/2

== system EV_basic_8_1/Vehicle components/Right Drive Inverter: Functional ==
  note: 3-Phase Inverter Output Current
  note: Inverter Input current
  note: Basic PWM controller for three phase current source inverter.
      | Inverter is operated to be always in-phase with rotor,
      | and control input sets the peak current of the produced
      | waveforms.
  note: Inverter Functional Model
  Vbus : Inport
  Fdrive_R : Inport  Port=2
  thetar : Inport  Port=3
  Pout : Inport  Port=4
  wr : Inport  Port=5
  Fv-to-Tm : Gain  Gain=rw/gratio
  Inverter Controller : Subsystem
  Inverter: Functional : Subsystem
  Motor Limits Model : Subsystem
  Saturation : Saturate  UpperLimit=3e5  LowerLimit=-3e5
  Iinv : Outport
  Iabc : Outport  Port=2
  wires:
  Inverter Controller/2(thetai) -> Inverter: Functional/1(thetai)
  Inverter Controller/1(Ipk) -> Inverter: Functional/2(Ipk)
  Inverter: Functional/2(Iinv) -> Iinv/1
  Inverter: Functional/1(Iabc) -> Iabc/1
  thetar/1 -> Inverter Controller/2(thetar)
  Pout/1 -> Saturation/1
  Vbus/1 -> Inverter: Functional/4(Vbus)
  Motor Limits Model/1(Tactual) -> Inverter Controller/1(Tactual)  "Tactual"
  wr/1 -> Motor Limits Model/1(wr)
  Fdrive_R/1 -> Fv-to-Tm/1
  Fv-to-Tm/1 -> Motor Limits Model/2(Tmcommand)  "Tmcommand"
  Saturation/1 -> Inverter: Functional/3(Pout)

== system EV_basic_8_1/Vehicle components/Subsystem ==
  VoltCmd : Inport
  SrcVolt : Inport  Port=2
  LdCurr : Inport  Port=3
  Add : Sum
  Add1 : Sum
  Bidirectional DC-DC : autolibdcdc/Bidirectional DC-DC  Tc=1/10  Vinit=Vbus_ref  Plimit=3e5  param_loss=Single efficiency measurement  eff=98  v_loss_bp=[0 200 400 600 800 1000]  i_loss_bp=[0 25 50 75 100]  losses_table=[100 100 100 100 100;100 150 200 250 300;100 200 300 400 500;100 250 400 550 700;100 300 500 700 900;100 350 600 850 1100]  v_eff_bp=[200 400 600 800 1000]  i_eff_bp=[25 50 75 100]  efficiency_table=[96.2 98.1 98.7 99;98.1 99 99.4 99.5;98.7 99.4 99.6 99.7;99 99.5 99.7 99.8;99.2 99.6 99.7 99.8]  x_v_bp=[-1000 -800 -600 -400 -200 200 400 600 800 1000]  x_i_bp=[-100 -75 -50 -25 25 50 75 100]  x_losses_mat=[200.400801603196 225.67703109328 200.803212851408 201.612903225806 199.999999999997 200 225 200;160.320641282556 180.541624874624 201.005025125625 202.020202020203 200 200 180 160;180.541624874624 180.722891566267 181.086519114686 197.568389057748 194.999999999999 179.999999999997 180 180;201.005025125625 181.086519114686 202.020202020203 193.67991845056 190 200 179.999999999997 200;202.020202020203 197.568389057748 193.67991845056 197.505197505197 190 190 194.999999999999 200;200 194.999999999999 190 190 197.505197505197 193.67991845056 197.568389057748 202.020202020203;200 179.999999999997 200 190 193.67991845056 202.020202020203 181.086519114686 201.005025125625;180 180 179.999999999997 194.999999999999 197.568389057748 181.086519114686 180.722891566267 180.541624874624;160 180 200 200 202.020202020203 201.005025125625 180.541624874624 160.320641282556;200 225 200 199.999999999997 201.612903225806 200.803212851408 225.67703109328 200.400801603196]
      settings: SourceProductName=Powertrain Blockset  SourceProductBaseCode=PW
  Constant : Constant  Value=0.02
  DC-DC Converter: Functional : Subsystem  Commented=on
      mask Display: image(imread('DC-DC.jpg'))
  Product : Product  Inputs=3
  Scope : Scope  NumInputPorts=2
  To Workspace : ToWorkspace  VariableName=dcdc_losses  SaveFormat=Structure With Time  SampleTime=s_time
  LdVolt : Outport
  SrcCurr : Outport  Port=2
  dcdc_losses : Outport  Port=3
  wires:
  VoltCmd/1 -> DC-DC Converter: Functional/1(Vref), Bidirectional DC-DC/1
  SrcVolt/1 -> Bidirectional DC-DC/2, DC-DC Converter: Functional/2(Vbat)
  LdCurr/1 -> Product/2, Bidirectional DC-DC/3, DC-DC Converter: Functional/3(Iout)
  Bidirectional DC-DC/2 -> Add/2, Product/1  "DC Bus Voltage"
  Bidirectional DC-DC/3 -> Add1/2  "Battery Current"
  Add/1 -> Scope/1, LdVolt/1
  Add1/1 -> Scope/2, SrcCurr/1
  DC-DC Converter: Functional/1(Vbus) -> Add/1  "DC Bus Voltage"
  DC-DC Converter: Functional/2(Ibat) -> Add1/1  "Battery Current"
  Constant/1 -> Product/3
  Product/1 -> dcdc_losses/1, To Workspace/1
